simulink model "model2"  (R2023a)
settings: Solver=ode4  StartTime=0.0  StopTime=10.0  FixedStep=1/216000  RelTol=1e-3
libraries: simulink x1
settings Model: Creator=tnt4  LastModifiedBy=tnt4
settings RTWCC: GPUComputeCapability=5.0

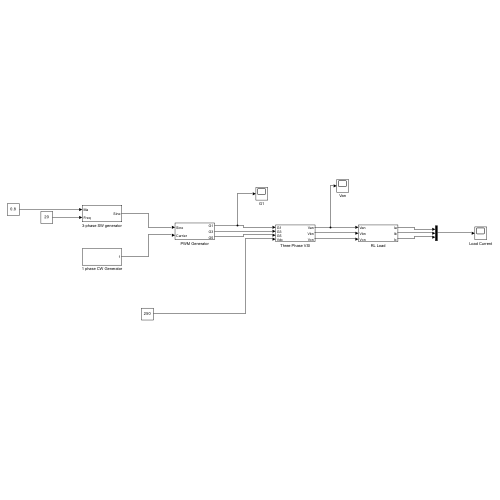
[thumbnail: Simulink's stored preview of the top-level diagram]
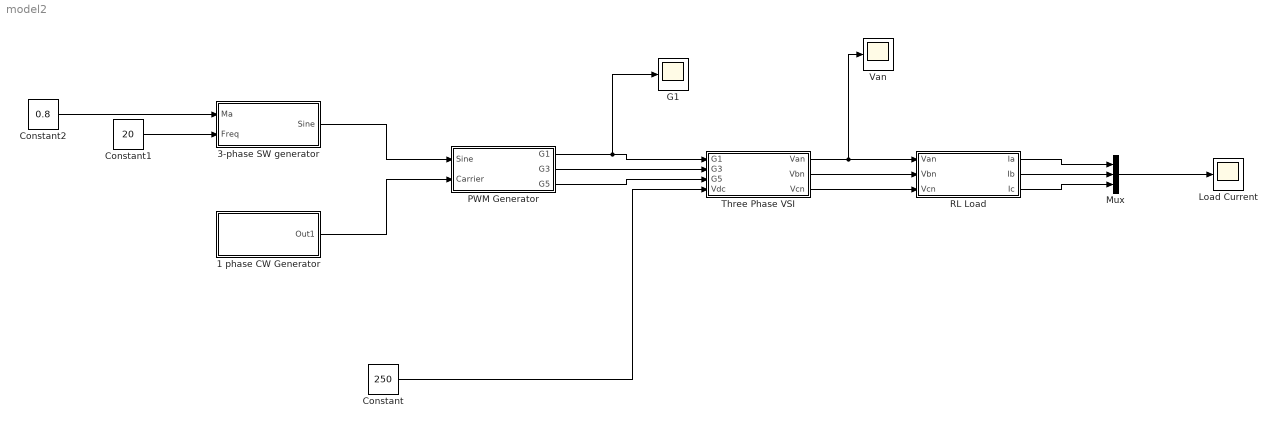
== system model2 ==
  1 phase CW Generator : Subsystem  mask{fc=240}
      mask prompts: fc "Carrier Frequency"
  3-phase SW generator : Subsystem
  Constant : Constant  Value=250
  Constant1 : Constant  Value=20
  Constant2 : Constant  Value=0.8
  G1 : Scope
  Load Current : Scope
  Mux : Mux  Inputs=3
  PWM Generator : Subsystem
  RL Load : Subsystem  mask{R_load=5, L_load=0.05}
      mask prompts: R_load "Resistance"; L_load "Inductance"
  Three Phase VSI : Subsystem
  Van : Scope
  wires:
  PWM Generator/1(G1) -> G1/1, Three Phase VSI/1(G1)
  PWM Generator/3(G5) -> Three Phase VSI/3(G5)
  PWM Generator/2(G3) -> Three Phase VSI/2(G3)
  Constant/1 -> Three Phase VSI/4(Vdc)
  Three Phase VSI/1(Van) -> Van/1, RL Load/1(Van)
  Three Phase VSI/2(Vbn) -> RL Load/2(Vbn)
  Three Phase VSI/3(Vcn) -> RL Load/3(Vcn)
  RL Load/1(Ia) -> Mux/1
  RL Load/2(Ib) -> Mux/2
  RL Load/3(Ic) -> Mux/3
  Mux/1 -> Load Current/1
  3-phase SW generator/1(Sine) -> PWM Generator/1(Sine)
  Constant1/1 -> 3-phase SW generator/2(Freq)
  Constant2/1 -> 3-phase SW generator/1(Ma)
  1 phase CW Generator/1(Out1) -> PWM Generator/2(Carrier)

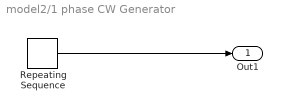
== system model2/1 phase CW Generator ==
  Repeating Sequence : simulink/Sources/Repeating Sequence  rep_seq_t=[0 1/(2*fc) 1/fc]  rep_seq_y=[-1 1 -1]
  Out1 : Outport
  wires:
  Repeating Sequence/1 -> Out1/1

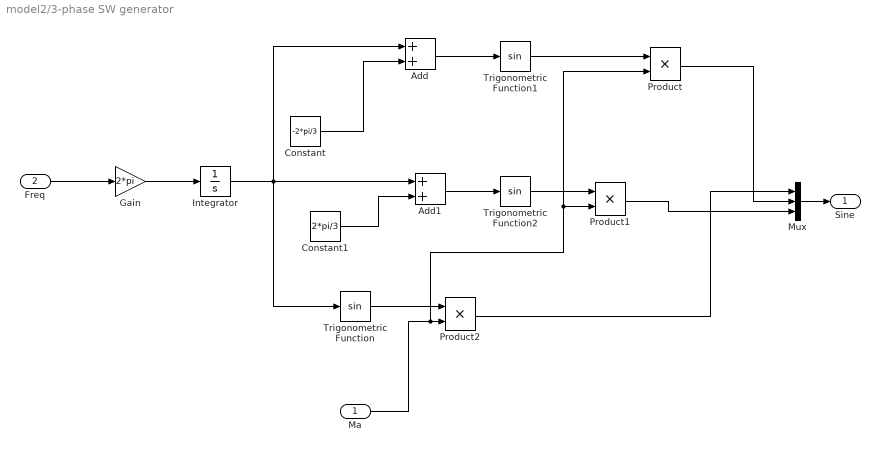
== system model2/3-phase SW generator ==
  Ma : Inport
  Freq : Inport  Port=2
  Add : Sum
  Add1 : Sum
  Constant : Constant  Value=-2*pi/3
  Constant1 : Constant  Value=2*pi/3
  Gain : Gain  Gain=2*pi
  Integrator : Integrator
  Mux : Mux  Inputs=3
  Product : Product
  Product1 : Product
  Product2 : Product
  Trigonometric Function : Trigonometry
  Trigonometric Function1 : Trigonometry
  Trigonometric Function2 : Trigonometry
  Sine : Outport
  wires:
  Freq/1 -> Gain/1
  Gain/1 -> Integrator/1
  Integrator/1 -> Add1/1, Add/1, Trigonometric Function/1
  Constant/1 -> Add/2
  Constant1/1 -> Add1/2
  Add/1 -> Trigonometric Function1/1
  Add1/1 -> Trigonometric Function2/1
  Trigonometric Function1/1 -> Product/1
  Trigonometric Function2/1 -> Product1/1
  Trigonometric Function/1 -> Product2/1
  Ma/1 -> Product1/2, Product/2, Product2/2
  Mux/1 -> Sine/1
  Product2/1 -> Mux/1
  Product/1 -> Mux/2
  Product1/1 -> Mux/3

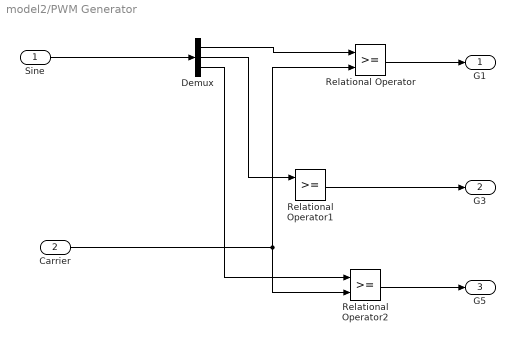
== system model2/PWM Generator ==
  Sine : Inport
  Carrier : Inport  Port=2
  Demux : Demux  Outputs=3
  Relational Operator : RelationalOperator  OutDataTypeStr=boolean  RndMeth=Simplest  InputSameDT=off
  Relational Operator1 : RelationalOperator  OutDataTypeStr=boolean  RndMeth=Simplest  InputSameDT=off
  Relational Operator2 : RelationalOperator  OutDataTypeStr=boolean  RndMeth=Simplest  InputSameDT=off
  G1 : Outport
  G3 : Outport  Port=2
  G5 : Outport  Port=3
  wires:
  Sine/1 -> Demux/1
  Demux/1 -> Relational Operator/1
  Demux/2 -> Relational Operator1/1
  Carrier/1 -> Relational Operator2/2, Relational Operator/2
  Demux/3 -> Relational Operator2/1
  Relational Operator/1 -> G1/1
  Relational Operator1/1 -> G3/1
  Relational Operator2/1 -> G5/1

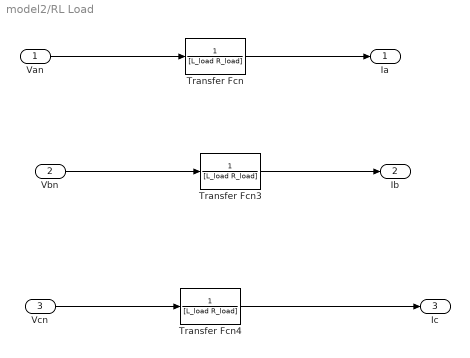
== system model2/RL Load ==
  Van : Inport
  Vbn : Inport  Port=2
  Vcn : Inport  Port=3
  Transfer Fcn : TransferFcn  Denominator=[L_load R_load]
  Transfer Fcn3 : TransferFcn  Denominator=[L_load R_load]
  Transfer Fcn4 : TransferFcn  Denominator=[L_load R_load]
  Ia : Outport
  Ib : Outport  Port=2
  Ic : Outport  Port=3
  wires:
  Transfer Fcn/1 -> Ia/1
  Van/1 -> Transfer Fcn/1
  Transfer Fcn3/1 -> Ib/1
  Vbn/1 -> Transfer Fcn3/1
  Vcn/1 -> Transfer Fcn4/1
  Transfer Fcn4/1 -> Ic/1

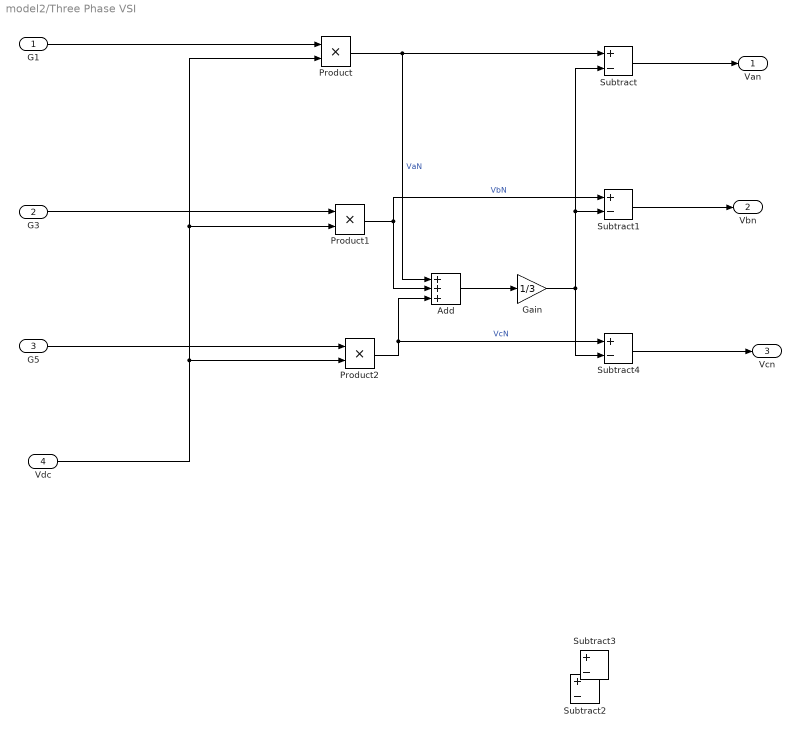
== system model2/Three Phase VSI ==
  G1 : Inport
  G3 : Inport  Port=2
  G5 : Inport  Port=3
  Vdc : Inport  Port=4
  Add : Sum  Inputs=+++
  Gain : Gain  Gain=1/3
  Product : Product
  Product1 : Product
  Product2 : Product
  Subtract{,1..4} (5 alike) : Sum  Inputs=+-
  Van : Outport
  Vbn : Outport  Port=2
  Vcn : Outport  Port=3
  wires:
  G1/1 -> Product/1
  G3/1 -> Product1/1
  G5/1 -> Product2/1
  Vdc/1 -> Product2/2, Product1/2, Product/2
  Product/1 -> Subtract/1, Add/1  "VaN"
  Product1/1 -> Add/2, Subtract1/1  "VbN"
  Product2/1 -> Add/3, Subtract4/1  "VcN"
  Add/1 -> Gain/1
  Gain/1 -> Subtract4/2, Subtract1/2, Subtract/2
  Subtract/1 -> Van/1
  Subtract1/1 -> Vbn/1
  Subtract4/1 -> Vcn/1
